simulink model "Fig4"  (R2015a)
settings: Solver=ode45  StartTime=0.0  StopTime=10.0  RelTol=1e-3
libraries: dspvision x1, dspsrcs4 x1, simulink x1, dspsnks4 x1, dspsigops x1
settings Model: Creator=Meghna  LastModifiedBy=Meghna

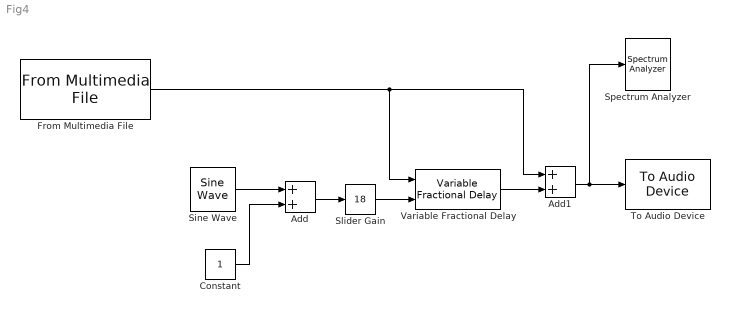
== system Fig4 ==
  Add : Sum
  Add1 : Sum
  Constant : Constant  SampleTime=1
  From Multimedia File : dspvision/From Multimedia File  inputFilename=speech_dft.mp3  loop=on  numPlays=inf  outputStreams=Audio only  videoDataType=single  audioDataType=double  inheritSampleTime=off  userDefinedSampleTime=1  noAudioOutput=off  isIntensityVideo=off  fourcc=RGB  colorVideoFormat=Separate color signals  outputEOF=off  dataOrg=Column-major  audioFrameSize=1536  computeAudioFrameSize=off  outSamplingMode=Sample based
  Sine Wave : dspsrcs4/Sine Wave  Amplitude=1  Frequency=100  Phase=0  SampleMode=Discrete  OutComplex=Real  CompMethod=Trigonometric fcn  TableSize=Speed  SampleTime=1  SamplesPerFrame=1  ResetState=Restart at time zero  dataType=double  wordLen=16  udDataType=sfix(16)  fracBitsMode=Best precision  numFracBits=15  OutDataTypeStr=double  LastOutDataTypeStr=double
  Slider Gain : simulink/Math Operations/Slider Gain  low=0  gain=18  high=36
  Spectrum Analyzer : SpectrumAnalyzer
  To Audio Device : dspsnks4/To Audio Device  deviceName=Default  inheritSampleRate=on  sampleRate=44100  deviceDatatype=Determine from input data type  autoBufferSize=on  bufferSize=4096  queueDuration=1.0  defaultOutputChannelMapping=on  outputChannelMapping=1:2  outputNumUnderrunSamples=off
  Variable Fractional Delay : dspsigops/Variable Fractional Delay  mode=OBSOLETE  modeActive=Linear  dmax=100  InputProcessing=Columns as channels (frame based)  L=4  FarrowL=4  R=10  alpha=1  ic=0  fallbackFIR=Clip to the minimum value necessary for centered kernel  fallbackFarrow=Clip to the minimum value necessary for centered kernel  noDFT=off  roundingMode=Zero  overflowMode=on
  wires:
  Sine Wave/1 -> Add/1
  Constant/1 -> Add/2
  From Multimedia File/1 -> Add1/1, Variable Fractional Delay/1
  Slider Gain/1 -> Variable Fractional Delay/2
  Add/1 -> Slider Gain/1
  Variable Fractional Delay/1 -> Add1/2
  Add1/1 -> Spectrum Analyzer/1, To Audio Device/1
